simulink model "Model_XStest"  (R2022a)
settings: Solver=VariableStepAuto  StartTime=6.69  StopTime=11.57  FixedStep=0.056  MaxStep=0.001  RelTol=1e-3  AbsTol=1e-3  EnableMultiTasking=on
values from neighbouring files (symbols this model uses):
  F = ec1807kf(ndx, 6)    [ga_optim.m]
  Sd = interp1(t, Sd, Tt1)    [ga_optim.m]
  V = ec1807k(ndx, 6)    [ga_optim.m]
  Xd = interp1(t, Xd, Tt1)    [ga_optim.m]
settings Model: ExtModeTrigMode=oneshot  ExtModeArmWhenConnect=off  Creator=Olympia  LastModifiedBy=Olympia
settings SolverCC: AutoScaleAbsTol=off  AlgebraicLoopSolver=TrustRegion
settings DataIOCC: SaveFormat=Array  SignalLoggingSaveFormat=ModelDataLogs  SaveOutput=off  SaveTime=off  ReturnWorkspaceOutputs=off
settings OptimizationCC: BlockReduction=off  BooleanDataType=off  ExpressionDepthLimit=2147483647  InitFltsAndDblsToZero=on  LifeSpan=inf
settings DebuggingCC: SaveWithParameterizedLinksMsg=none  UnderspecifiedInitializationDetection=Classic  MergeDetectMultiDrivingBlocksExec=none  SignalResolutionControl=TryResolveAllWithWarning  MultiTaskDSMMsg=warning  MultiTaskCondExecSysMsg=none  FcnCallInpInsideContextMsg=warning  UnconnectedInputMsg=warning  UnconnectedOutputMsg=warning  UnconnectedLineMsg=warning  StateNameClashWarn=warning  SFUnexpectedBacktrackingDiag=warning  SFNoUnconditionalDefaultTransitionDiag=warning  SFExecutionAtInitializationDiag=none  SFMachineParentedDataDiag=warning  ArithmeticOperatorsInVariantConditions=warning
settings HardwareCC: ProdBitPerPointer=32  ProdBitPerSizeT=32  ProdBitPerPtrDiffT=32  ProdLargestAtomicFloat=None  ProdIntDivRoundTo=Undefined  ProdEndianess=Unspecified  ProdWordSize=32  ProdHWDeviceType=32-bit Generic  TargetUnknown=on
settings ModelReferenceCC: PropagateSignalLabelsOutOfModel=off
settings SFSimCC: SimUseLocalCustomCode=off  CustomCodeUndefinedFunction=UseInterfaceOnly
settings RTWCC: RTWUseLocalCustomCode=off
settings CodeAppCC: StateflowObjectComments=on
settings GRTTargetCC: TargetLangStandard=C89/C90 (ANSI)  ModelReferenceCompliant=off  CompOptLevelCompliant=off  CombineOutputUpdateFcns=off  MatFileLogging=off  GRTInterface=on
settings ConfigComp: CovMetricSettings=dw  CovSaveCumulativeToWorkspaceVar=on  CovSaveSingleToWorkspaceVar=on  CovExternalEMLEnable=off

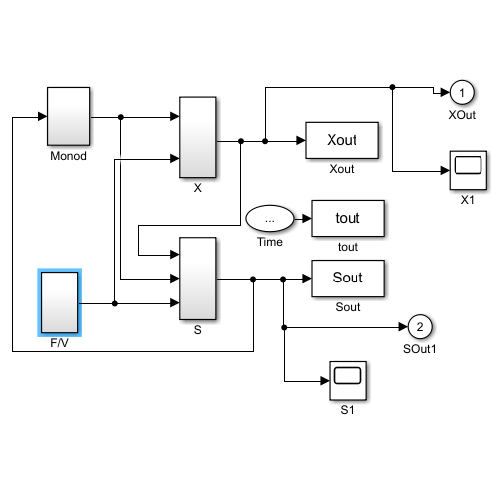
[thumbnail: Simulink's stored preview of the top-level diagram]
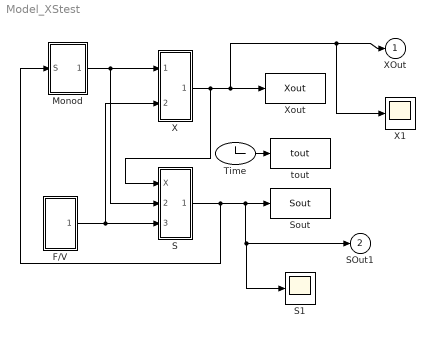
== system Model_XStest ==
  F/V : Subsystem
  Monod : Subsystem
  S : Subsystem
  S1 : Scope
  Sout : ToWorkspace  VariableName=Sout  SampleTime=-1
  Time : Clock
  X : Subsystem
  X1 : Scope
  Xout : ToWorkspace  VariableName=Xout  SampleTime=-1
  tout : ToWorkspace  VariableName=tout  SampleTime=-1
  XOut : Outport
  SOut1 : Outport  Port=2
  wires:
  X/1(XOut) -> S/1(X), Xout/1, X1/1, XOut/1
  S/1(Sout) -> Monod/1(S), Sout/1, S1/1, SOut1/1
  Time/1 -> tout/1
  F/V/1(out_1) -> S/3(F/V), X/2(F/V)
  Monod/1(mu) -> X/1(mu), S/2(mu)

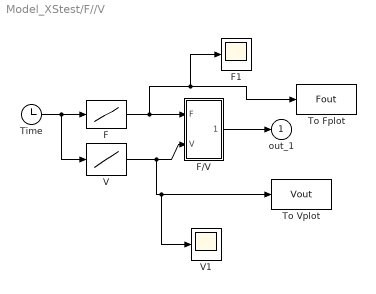
== system Model_XStest/F//V ==
  F : Lookup  InputValues=t  Table=F
  F/V : Subsystem  mask(/){}
      mask help: Division of two scalars. y=u[1]/u[2]
      mask Help: Division of two scalars: y=u[1]/u[2]
      mask Display: disp('/')
  F1 : Scope
  Time : Clock
  To Fplot : ToWorkspace  VariableName=Fout  SampleTime=-1
  To Vplot : ToWorkspace  VariableName=Vout  SampleTime=-1
  V : Lookup  InputValues=t  Table=V
  V1 : Scope
  out_1 : Outport
  wires:
  F/V/1(out_1) -> out_1/1
  F/1 -> F1/1, To Fplot/1, F/V/1(F)
  V/1 -> V1/1, To Vplot/1, F/V/2(V)
  Time/1 -> F/1, V/1

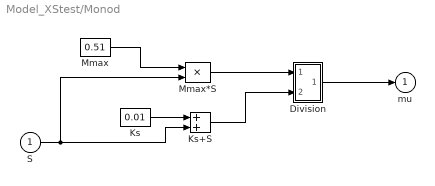
== system Model_XStest/Monod ==
  S : Inport
  Division : Subsystem  mask(/){}
      mask help: Division of two scalars. y=u[1]/u[2]
      mask Help: Division of two scalars: y=u[1]/u[2]
      mask Display: disp('/')
  Ks : Constant  Value=0.01
  Ks+S : Sum  InputSameDT=on  SaturateOnIntegerOverflow=on  OutDataTypeStr=Inherit: Same as first input
  Mmax : Constant  Value=0.51
  Mmax*S : Product  InputSameDT=on  RndMeth=Zero  SaturateOnIntegerOverflow=on  OutDataTypeStr=Inherit: Same as first input
  mu : Outport
  wires:
  Division/1(out_1) -> mu/1
  Mmax/1 -> Mmax*S/1
  Mmax*S/1 -> Division/1(Mmax*S)
  Ks+S/1 -> Division/2(Ks+S)
  Ks/1 -> Ks+S/1
  S/1 -> Ks+S/2, Mmax*S/2

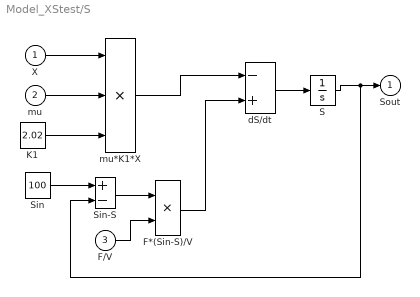
== system Model_XStest/S ==
  X : Inport
  mu : Inport  Port=2
  F/V : Inport  Port=3
  F*(Sin-S)/V : Product  InputSameDT=on  RndMeth=Zero  SaturateOnIntegerOverflow=on  OutDataTypeStr=Inherit: Same as first input
  K1 : Constant  Value=2.02
  S : Integrator  InitialCondition=Sd(1)  UpperSaturationLimit=1000  LowerSaturationLimit=0
  Sin : Constant  Value=100
  Sin-S : Sum  Inputs=+-  InputSameDT=on  SaturateOnIntegerOverflow=on  OutDataTypeStr=Inherit: Same as first input
  dS/dt : Sum  Inputs=-+  InputSameDT=on  SaturateOnIntegerOverflow=on  OutDataTypeStr=Inherit: Same as first input
  mu*K1*X : Product  Inputs=3  InputSameDT=on  RndMeth=Zero  SaturateOnIntegerOverflow=on  OutDataTypeStr=Inherit: Same as first input
  Sout : Outport
  wires:
  S/1 -> Sout/1, Sin-S/2
  Sin-S/1 -> F*(Sin-S)/V/1
  Sin/1 -> Sin-S/1
  X/1 -> mu*K1*X/1
  F/V/1 -> F*(Sin-S)/V/2
  mu*K1*X/1 -> dS/dt/1
  F*(Sin-S)/V/1 -> dS/dt/2
  dS/dt/1 -> S/1
  mu/1 -> mu*K1*X/2
  K1/1 -> mu*K1*X/3

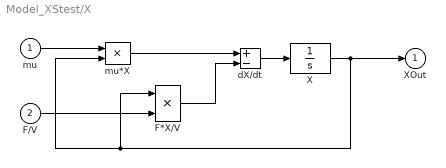
== system Model_XStest/X ==
  mu : Inport
  F/V : Inport  Port=2
  F*X/V : Product  InputSameDT=on  RndMeth=Zero  SaturateOnIntegerOverflow=on  OutDataTypeStr=Inherit: Same as first input
  X : Integrator  InitialCondition=Xd(1)  UpperSaturationLimit=1000  LowerSaturationLimit=0
  dX/dt : Sum  Inputs=+-  InputSameDT=on  SaturateOnIntegerOverflow=on  OutDataTypeStr=Inherit: Same as first input
  mu*X : Product  InputSameDT=on  RndMeth=Zero  SaturateOnIntegerOverflow=on  OutDataTypeStr=Inherit: Same as first input
  XOut : Outport
  wires:
  F*X/V/1 -> dX/dt/2
  dX/dt/1 -> X/1
  mu*X/1 -> dX/dt/1
  mu/1 -> mu*X/1
  X/1 -> XOut/1, mu*X/2, F*X/V/1
  F/V/1 -> F*X/V/2

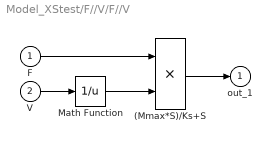
== system Model_XStest/F//V/F//V ==
  F : Inport
  V : Inport  Port=2
  (Mmax*S)/Ks+S : Product  InputSameDT=on  RndMeth=Zero  SaturateOnIntegerOverflow=on  OutDataTypeStr=Inherit: Same as first input
  Math Function : Math  Operator=reciprocal  SignedPower=on
  out_1 : Outport
  wires:
  F/1 -> (Mmax*S)/Ks+S/1
  V/1 -> Math Function/1
  Math Function/1 -> (Mmax*S)/Ks+S/2
  (Mmax*S)/Ks+S/1 -> out_1/1

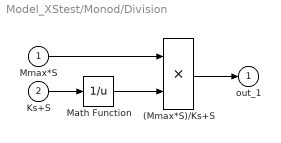
== system Model_XStest/Monod/Division ==
  Mmax*S : Inport
  Ks+S : Inport  Port=2
  (Mmax*S)/Ks+S : Product  InputSameDT=on  RndMeth=Zero  SaturateOnIntegerOverflow=on  OutDataTypeStr=Inherit: Same as first input
  Math Function : Math  Operator=reciprocal  SignedPower=on
  out_1 : Outport
  wires:
  Mmax*S/1 -> (Mmax*S)/Ks+S/1
  Ks+S/1 -> Math Function/1
  Math Function/1 -> (Mmax*S)/Ks+S/2
  (Mmax*S)/Ks+S/1 -> out_1/1
